simulink model "quadcopter_model"  (R2020b)
settings: Solver=VariableStepAuto  StartTime=0.0  StopTime=10  RelTol=1e-3
values from neighbouring files (symbols this model uses):
  h_des = 1    [main_quadcopter_sim.m]
  K_z = 6.0    (= 6)    [main_quadcopter_sim.m]
  quad_data = [   9.81,   0.063,  5.82857e-05,   7.16914e-05,   1.0e-04,       0.0624,       0.0107,       7.8264e-04,   1.15         ]    [main_quadcopter_sim.m]
  y_init_conds = [ ... (first row only)    [main_quadcopter_sim.m]
undefined symbols (not defined in the file or in its folder): KD_z, KI_z, KP_z
libraries: pid_lib x1
settings Model: Creator=kekko  LastModifiedBy=kekko

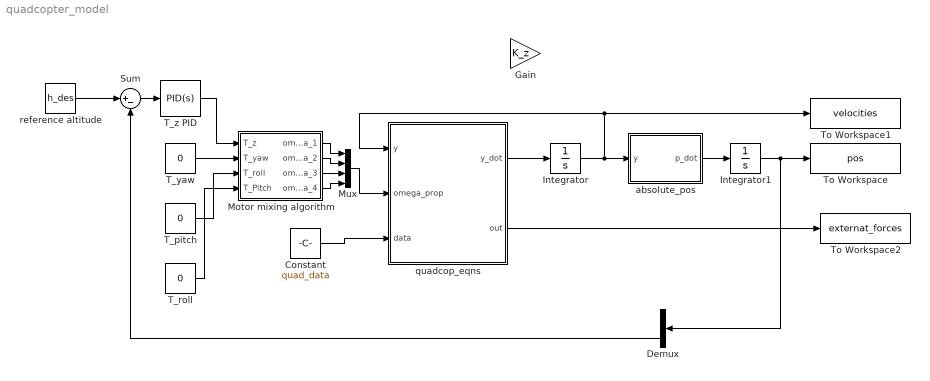
== system quadcopter_model ==
  Constant : Constant  Value=quad_data
  Demux : Demux  Outputs=3
  Gain : Gain  Gain=K_z
  Integrator : Integrator  InitialCondition=y_init_conds
  Integrator1 : Integrator  InitialCondition=[0 0 0]
  Motor mixing algorithm : Subsystem
  Mux : Mux
  Sum : Sum  Inputs=|+-
  T_pitch : Constant  Value=0
  T_roll : Constant  Value=0
  T_yaw : Constant  Value=0
  T_z PID : pid_lib/PID Controller  Controller=PID  Form=Parallel  TimeDomain=Continuous-time  UseExternalTs=off  SampleTime=-1  IntegratorMethod=Forward Euler  FilterMethod=Forward Euler  ControllerParametersSource=internal  P=KP_z  I=KI_z  D=KD_z  UseFilter=on  N=100  TunerSelectOption=Transfer Function Based (PID Tuner App)  InitialConditionSource=internal  InitialConditionForIntegrator=0  InitialConditionForFilter=0  DifferentiatorICPrevScaledInput=0  ExternalReset=none  TrackingMode=off  Kt=1  LimitOutput=off  SatLimitsSource=internal  UpperSaturationLimit=inf  LowerSaturationLimit=-inf  LinearizeAsGain=on  AntiWindupMode=none  Kb=1  POutMin=[]  POutMax=[]  IOutMin=[]  IOutMax=[]  DOutMin=[]  DOutMax=[]  NOutMin=[]  NOutMax=[]  SumOutMin=[]  SumOutMax=[]  SaturationOutMin=[]  SaturationOutMax=[]  PParamMin=[]  PParamMax=[]  IParamMin=[]  IParamMax=[]  DParamMin=[]  DParamMax=[]  NParamMin=[]  NParamMax=[]  KbParamMin=[]  KbParamMax=[]  KtParamMin=[]  KtParamMax=[]  KbOutMin=[]  KbOutMax=[]  KtOutMin=[]  KtOutMax=[]  IntegratorOutMin=[]  IntegratorOutMax=[]  FilterOutMin=[]  FilterOutMax=[]  SumI1OutMin=[]  SumI1OutMax=[]  SumI2OutMin=[]  SumI2OutMax=[]  SumI3OutMin=[]  SumI3OutMax=[]  SumI4OutMin=[]  SumI4OutMax=[]  SumDOutMin=[]  SumDOutMax=[]  DifferentiatorOutMin=[]  DifferentiatorOutMax=[]  FilterDiffOutCoefMin=[]  FilterDiffOutCoefMax=[]  ReciprocalOutMin=[]  ReciprocalOutMax=[]  SumDenOutMin=[]  SumDenOutMax=[]  SumNumOutMin=[]  SumNumOutMax=[]  DivideOutMin=[]  DivideOutMax=[]  UdiffTsProdOutMin=[]  UdiffTsProdOutMax=[]  NTsProdOutMin=[]  NTsProdOutMax=[]  UintegralTsProdOutMin=[]  UintegralTsProdOutMax=[]  UngainTsProdOutMin=[]  UngainTsProdOutMax=[]  IntegratorContinuousStateAttributes=''  IntegratorStateMustResolveToSignalObject=off  IntegratorRTWStateStorageClass=Auto  FilterContinuousStateAttributes=''  FilterStateMustResolveToSignalObject=off  FilterRTWStateStorageClass=Auto  ParallelPVariant=InternalParameters  IdealPVariant=Disabled  IVariant=InternalParameters  DVariant=InternalParameters  IntegratorVariant=Continuous  SatVariant=Disabled  AWVariant=Passthrough  PCopyVariant=Disabled  TRVariant=Disabled  FdbkBlocksVariant=Forward  IdealPFdbkVariant=Disabled  SatFdbkVariant=Disabled  DerivativeFilterVariant=ContFilter  NVariant=InternalParameters  NCopyVariant=Disabled  FilterICVariant=InternalICsFilter  IntegratorICVariant=InternalICs  ExternalResetVariant=Disabled  TRSumVariant=Passthrough  SumFdbkVariant=Disabled  SumVariant=Sum_PID  TsampFilterVariant=InternalTs  TsampNgainVariant=Passthrough  TsampIntegralVariant=Passthrough  ExternalSaturationOutDataTypeStr=Inherit: Same as second input
  To Workspace : ToWorkspace  VariableName=pos  SampleTime=-1
      settings: Save2DSignal=2-D array (concatenate along first dimension)
  To Workspace1 : ToWorkspace  VariableName=velocities  SampleTime=-1
      settings: Save2DSignal=2-D array (concatenate along first dimension)
  To Workspace2 : ToWorkspace  VariableName=externat_forces  SampleTime=-1
      settings: Save2DSignal=2-D array (concatenate along first dimension)
  absolute_pos : MATLAB Function  TreatAsAtomicUnit=on
  quadcop_eqns : MATLAB Function  TreatAsAtomicUnit=on
  reference altitude : Constant  Value=h_des
  wires:
  Constant/1 -> quadcop_eqns/3(data)
  quadcop_eqns/1(y_dot) -> Integrator/1
  Integrator/1 -> absolute_pos/1(y), To Workspace1/1, quadcop_eqns/1(y)
  absolute_pos/1(p_dot) -> Integrator1/1
  Integrator1/1 -> To Workspace/1, Demux/1
  quadcop_eqns/2(out) -> To Workspace2/1
  Mux/1 -> quadcop_eqns/2(omega_prop)
  Demux/3 -> Sum/2
  reference altitude/1 -> Sum/1
  Sum/1 -> T_z PID/1
  T_z PID/1 -> Motor mixing algorithm/1(T_z)
  Motor mixing algorithm/4(omega_4) -> Mux/4
  T_yaw/1 -> Motor mixing algorithm/2(T_yaw)
  T_pitch/1 -> Motor mixing algorithm/3(T_roll)
  T_roll/1 -> Motor mixing algorithm/4(T_Pitch)
  Motor mixing algorithm/1(omega_1) -> Mux/1
  Motor mixing algorithm/2(omega_2) -> Mux/2
  Motor mixing algorithm/3(omega_3) -> Mux/3

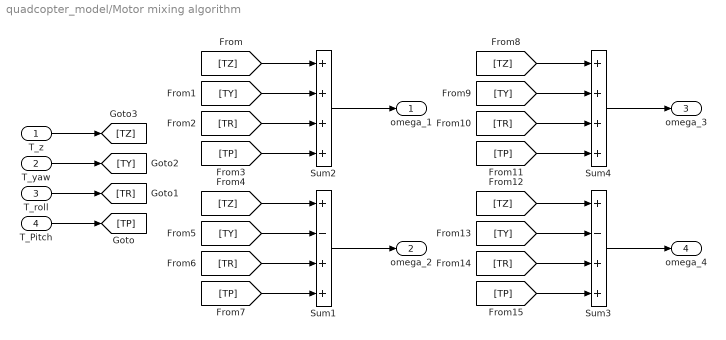
== system quadcopter_model/Motor mixing algorithm ==
  T_z : Inport
  T_yaw : Inport  Port=2
  T_roll : Inport  Port=3
  T_Pitch : Inport  Port=4
  Sum1 : Sum  Inputs=+-++
  Sum2 : Sum  Inputs=++++
  Sum3 : Sum  Inputs=+-++
  Sum4 : Sum  Inputs=++++
  omega_1 : Outport
  omega_2 : Outport  Port=2
  omega_3 : Outport  Port=3
  omega_4 : Outport  Port=4
  wires:
  Sum2/1 -> omega_1/1
  T_Pitch/1 -> [TP]
  T_roll/1 -> [TR]
  T_yaw/1 -> [TY]
  T_z/1 -> [TZ]
  [TZ] -> Sum2/1
  [TY] -> Sum2/2
  [TR] -> Sum2/3
  [TP] -> Sum2/4
  Sum1/1 -> omega_2/1
  [TZ] -> Sum1/1
  [TP] -> Sum1/4
  [TR] -> Sum1/3
  [TY] -> Sum1/2
  Sum4/1 -> omega_3/1
  [TZ] -> Sum4/1
  [TP] -> Sum4/4
  [TZ] -> Sum3/1
  [TP] -> Sum3/4
  [TY] -> Sum3/2
  [TR] -> Sum3/3
  [TR] -> Sum4/3
  Sum3/1 -> omega_4/1
  [TY] -> Sum4/2

== matlab function quadcopter_model/absolute_pos ==
  data: y input; p_dot output
function p_dot = fcn(y)
  
  % remapping ============================
  u       = y(1);
  v       = y(2);
  w       = y(3);
  omega_x = y(4);
  omega_y = y(5);
  omega_z = y(6);
  phi     = y(7);
  theta   = y(8);
  psi     = y(9);
  
  % ode for absolute position (right hand side )
  p_dot = [ ((sin(phi) * v + w * cos(phi)) * sin(theta) + cos(theta) * u) * cos(psi) + sin(psi) * (sin(phi) * w - v * cos(phi)),...
            ((sin(phi) * v + w * cos(phi)) * sin(theta) + cos(theta) * u) * sin(psi) - cos(psi) * (sin(phi) * w - v * cos(phi)),...
            w * cos(theta) * cos(phi) + v * cos(theta) * sin(phi) - u * sin(theta)...
         ];
end

== matlab function quadcopter_model/quadcop_eqns ==
  data: y input; y_dot output; omega_prop input; data input; out output
function [y_dot , out ] = fcn(y,omega_prop,data)
  % y' = y_dot = rhs(y,omega_prop)
  % y = [u,v,w,omega_x,omega_y,omega_z,phi,theta,psi]
  % y(1) = u ....
  
  % extract data from vector
  g = data(1);
  m = data(2);
  ixx = data(3);
  iyy = data(4);
  izz = data(5);
  L   = data(6);
  CT  = data(7);
  CQ  = data(8);
  rho = data(9);
  
  
  % remapping ============================
  u       = y(1);
  v       = y(2);
  w       = y(3);
  omega_x = y(4);
  omega_y = y(5);
  omega_z = y(6);
  phi     = y(7);
  theta   = y(8);
  psi     = y(9);
  % extract angular velocities of propeller
  omega1 = omega_prop(1);
  omega2 = omega_prop(2);
  omega3 = omega_prop(3);
  omega4 = omega_prop(4);
  
  % external force model ==================
  % thrust forces of propeller
  ft1 = rho*CT*omega1^2;
  ft2 = rho*CT*omega2^2;
  ft3 = rho*CT*omega3^2;
  ft4 = rho*CT*omega4^2;
  
  % drag torques of propeller
  tauD1 = +rho*CQ*omega1^2;
  tauD2 = -rho*CQ*omega2^2;
  tauD3 = +rho*CQ*omega3^2;
  tauD4 = -rho*CQ*omega4^2;
  
  % aerodynamic drag + wind
  % add later on ...
  
  % equations angular velocities 
  
  % rhs equations of NE ====================================
  y_dot = [sin(theta) * g + v * omega_z - w * omega_y,...
          -sin(phi) * cos(theta) * g - u * omega_z + w * omega_x ,...
          -0.1e1 / m * (cos(phi) * cos(theta) * g * m + v * omega_x * m - u * omega_y * m - ft1 - ft3 - ft4 - ft2),...
          (iyy - izz) * omega_z / ixx * omega_y - L * (ft2 - ft4) / ixx ,...
          (-ixx + izz) * omega_z / iyy * omega_x - L * (ft1 - ft3) / iyy,...
          (omega_y * (ixx - iyy) * omega_x + tauD1 + tauD2 + tauD3 + tauD4)/ izz,...
          (sin(theta) * omega_z * cos(phi) + sin(theta) * omega_y * sin(phi) + omega_x * cos(theta)) / cos(theta),...
          -omega_z * sin(phi) + omega_y * cos(phi),...
          (omega_z * cos(phi) + omega_y * sin(phi)) / cos(theta)];

  
%   y_dot = [...
%     omega_z*v-omega_y*w+sin(theta)*g, ...
%     -omega_z*u+w*omega_x-cos(theta)*sin(phi)*g, ...
%     -v*omega_x+u*omega_y+cos(phi)*cos(theta)*g+(ft1+ft2+ft3+ft4)/m,...
%     omega_z*omega_y*(iyy-izz)/ixx-L*(ft2-ft4)/ixx,...
%     -omega_z*omega_x*(ixx-izz)/iyy-L*(ft1-ft3)/iyy,...
%     omega_y*omega_x*(ixx-iyy)/izz+(tauD1+tauD2+tauD3+tauD4)/izz,...
%     -omega_x-sin(theta)*sin(phi)/cos(theta)*omega_y-sin(theta)*cos(phi)/cos(theta)*omega_z,...
%     -cos(phi)*omega_y+sin(phi)*omega_z,...
%     -sin(phi)/cos(theta)*omega_y-cos(phi)/cos(theta)*omega_z];
  
  % export values of external forces
  out = [ft1,ft2,ft3,ft4,tauD1,tauD2,tauD3,tauD4];

end
